simulink model "friction_Pcontrol"  (R2017a)
settings: Solver=ode4  StartTime=0.0  StopTime=80  FixedStep=1e-3  RelTol=1e-3
values from neighbouring files (symbols this model uses):
  ctrl_mass = mass    (= 3.14)    [Script_Friction.m]
  ctrl_ts = 1e-3    (= 0.001)    [Script_Friction.m]
  Fc = 2    [Script_Friction.m]
  Fs = 3    [Script_Friction.m]
  i = 2    [Script_Friction.m]
  kv = 1    [Script_Friction.m]
  m = 3.14    [Static_Identif.m]    (also in static_optim.m)
  mass = 8.1    [C_script_dyn_optimization.m]    (also in Script_Friction.m = 3.14; identify_dynamic_param.m)
  N = 100    [A_Static_Experiment.m]    (also in identify_static_param.m; obtain_sim_data.m = round(length(x) / 2); run_sim.m)
  ref_angle = 0.01    [run_sim.m]
  sigma0 = 1000    [Script_Friction.m]
  sigma1 = 200    [Script_Friction.m]
  sigma2 = 0.1    [C_script_dyn_optimization.m]    (also in Script_Friction.m = 1)
  tol_ss = ref_angle*5e-3    (= 5e-05)    [run_sim.m]
  ts_buffer_stop = ctrl_ts    (= 0.001)    [Script_Friction.m]
  vs = 0.01    [Script_Friction.m]
  X = otim    [A_Static_Experiment.m]    (also in Static_Identif.m = X + 1.0 * V; identify_static_param.m; interval_definition.m = sprintf('Data from interval; static_optim.m = X + 1.0 * V)
undefined symbols (not defined in the file or in its folder): Y, Z
libraries: simulink x11, sm_lib x8, nesl_utility x5, checkpacklib x2, fl_lib x2, Multibody_Multiphysics_Lib x1
settings Model: Creator=jcmonteiro  LastModifiedBy=igricart
settings DataIOCC: ReturnWorkspaceOutputs=on  ReturnWorkspaceOutputsName=SDOSimTest_Log

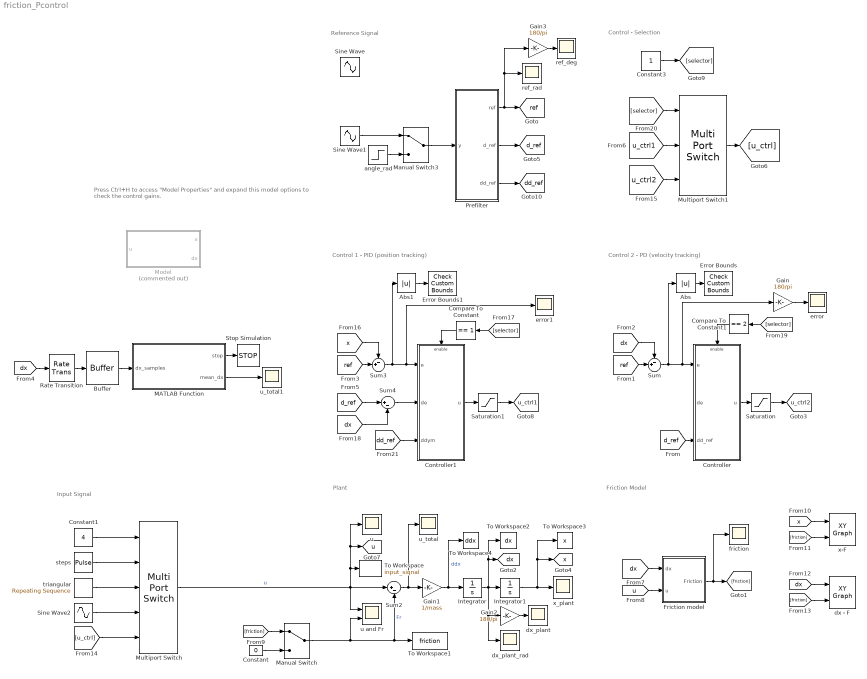
== system friction_Pcontrol ==
  note: Input Signal
  note: Control 2 - PD (velocity tracking)
  note: Plant
  note: Reference Signal
  note: Press Ctrl+H to access "Model Properties" and expand this model options
      | to check the control gains.
  note: Friction Model
  note: Control 1 - PID (position tracking)
  note: Control - Selection
  Abs : Abs
  Abs1 : Abs
  Buffer : Buffer  N=2/ts_buffer_stop  V=2/ts_buffer_stop - 1  ic=(tol_ss + 1) * ones(2/ts_buffer_stop,1)  OutputFrames=off
  Compare To Constant : simulink/Logic and Bit Operations/Compare To Constant  relop===  const=1  OutDataTypeStr=boolean
  Compare To Constant1 : simulink/Logic and Bit Operations/Compare To Constant  relop===  const=2  OutDataTypeStr=boolean
  Constant : Constant  Value=0
  Constant1 : Constant  Value=4
  Constant3 : Constant  OutMin=1  OutMax=2
  Controller : Subsystem  mask{wn=0.5, damp=0.95, far=3}
      mask prompts: wn "Natural frequency"; damp "Damping"; far "Far pole"
      mask init:
      | Kd = far + 2*damp*wn;
      | Kp = wn*wn + 2*damp*wn*far;
      | Ki = far*wn*wn;
  Controller1 : Subsystem  mask{wn=5, damp=0.95, far=2}
      mask prompts: wn "Natural frequency"; damp "Damping"; far "Far pole"
      mask init:
      | Kd = far + 2*damp*wn;
      | Kp = wn*wn + 2*damp*wn*far;
      | Ki = far*wn*wn;
  Error Bounds : checkpacklib/Check Custom Bounds  InstantiateOnLoad=on  enabled=off  stopWhenAssertionFail=off  export=off  ViewDlgPos=[224 43 510 418]  OpenViewOnLoad=off  LaunchViewOnOpen=off  TimeUnits=seconds  EnableUpperBound=on  UpperBoundTimes=[0 1; 1 4; 4 20]  UpperBoundAmplitudes=[4e-3 4e-3; 2e-3 2e-3; 3.5e-4 3.5e-4];  EnableLowerBound=off  LowerBoundTimes=[]  LowerBoundAmplitudes=[]
  Error Bounds1 : checkpacklib/Check Custom Bounds  InstantiateOnLoad=on  enabled=off  stopWhenAssertionFail=off  export=off  ViewDlgPos=[224 43 510 418]  OpenViewOnLoad=off  LaunchViewOnOpen=off  TimeUnits=seconds  EnableUpperBound=on  UpperBoundTimes=[0 1; 1 4; 4 20]  UpperBoundAmplitudes=[4e-3 4e-3; 2e-3 2e-3; 3.5e-4 3.5e-4];  EnableLowerBound=off  LowerBoundTimes=[]  LowerBoundAmplitudes=[]
  Friction model : Subsystem
  Gain : Gain  Gain=180/pi
  Gain1 : Gain  Gain=1/mass
  Gain2 : Gain  Gain=180/pi
  Gain3 : Gain  Gain=180/pi
  Integrator : Integrator
  Integrator1 : Integrator
  MATLAB Function : MATLAB Function  TreatAsAtomicUnit=on
  Manual Switch : ManualSwitch
  Manual Switch3 : ManualSwitch
  Model : Subsystem  Commented=on
  Multiport Switch : MultiPortSwitch  Inputs=4
  Multiport Switch1 : MultiPortSwitch  Inputs=2
  Prefilter : Subsystem  mask{refmodel_wn=6, refmodel_eta=1}
      mask prompts: refmodel_wn "Natural Frequency"; refmodel_eta "Damping"
      mask init:
      | refmodel_eta = abs(refmodel_eta);
      | refmodel_eta = min(refmodel_eta, 1);
      | 
      | refmodel_wn = abs(refmodel_wn);
  Rate Transition : RateTransition  OutPortSampleTime=ts_buffer_stop
  Saturation : Saturate  UpperLimit=20  LowerLimit=-20
  Saturation1 : Saturate  UpperLimit=20  LowerLimit=-20
  Sine Wave : Sin  Amplitude=ref_angle  Frequency=2*pi/1  SampleTime=ctrl_ts
  Sine Wave1 : Sin  Amplitude=0.01  Frequency=2*pi/4  SampleTime=0
  Sine Wave2 : Sin  Amplitude=2.8  Frequency=2*pi  SampleTime=ctrl_ts
  Stop Simulation : Stop
  Sum : Sum  Inputs=-+|
  Sum2 : Sum  Inputs=|+-
  Sum3 : Sum  Inputs=-+|
  Sum4 : Sum  Inputs=|+-
  To Workspace : ToWorkspace  VariableName=input_signal  SaveFormat=Structure With Time  SampleTime=-1
  To Workspace1 : ToWorkspace  VariableName=friction  SaveFormat=Structure With Time  SampleTime=-1
  To Workspace2 : ToWorkspace  VariableName=dx  SaveFormat=Structure With Time  SampleTime=-1
  To Workspace3 : ToWorkspace  VariableName=x  SaveFormat=Structure With Time  SampleTime=-1
  To Workspace4 : ToWorkspace  VariableName=ddx  SaveFormat=Structure With Time  SampleTime=-1
  angle_rad : Step  Time=0  After=ref_angle  SampleTime=0
  dx - F : simulink/Sinks/XY Graph  xmin=-0.6  xmax=0.6  ymin=-Fs*3  ymax=Fs*3  st=-1
  dx_plant : Scope
  dx_plant_rad : Scope
  error : Scope
  error1 : Scope
  friction : Scope
  ref_deg : Scope
  ref_rad : Scope
  steps : DiscretePulseGenerator  PulseType=Time based  Period=10  PulseWidth=5
  triangular : simulink/Sources/Repeating Sequence  rep_seq_t=[0 6]  rep_seq_y=[0 8]
  u : Scope
  u and Fr : Scope  NumInputPorts=2
  u_total : Scope
  u_total1 : Scope
  x-F : simulink/Sinks/XY Graph  xmin=-1e-3  xmax=10e-3  ymin=-Fs*1.2  ymax=Fs*1.2  st=-1
  x_plant : Scope
  tag scope: d_ref=global, dd_ref=global, dx=global, ref=global, u=global, u_ctrl1=global, u_ctrl2=global, x=global
  wires:
  Integrator1/1 -> x_plant/1, To Workspace3/1, [x]
  Integrator/1 -> Gain2/1, dx_plant_rad/1, Integrator1/1, To Workspace2/1, [dx]
  Gain1/1 -> To Workspace4/1, Integrator/1  "ddx"
  Manual Switch3/1 -> Prefilter/1(y)
  angle_rad/1 -> Manual Switch3/2
  Prefilter/1(ref) -> Gain3/1, ref_rad/1, [ref]
  Abs/1 -> Error Bounds/1
  Controller/1(u) -> Saturation/1
  Saturation/1 -> [u_ctrl2]
  Prefilter/2(d_ref) -> [d_ref]
  [d_ref] -> Controller/3(dd_ref)
  Sum/1 -> Abs/1, Gain/1, Controller/1(e)
  [ref] -> Sum/2
  [dx] -> Sum/1
  [dx] -> Friction model/1(dx)
  Sum2/1 -> Gain1/1, u_total/1
  [friction] -> Manual Switch/1
  Constant/1 -> Manual Switch/2
  Manual Switch/1 -> u and Fr/2, To Workspace1/1, Sum2/2  "Fr"
  [friction] -> x-F/2
  [x] -> x-F/1
  [dx] -> dx - F/1
  [friction] -> dx - F/2
  Friction model/1(Friction) -> friction/1, [friction]
  Multiport Switch/1 -> u/1, [u], To Workspace/1, u and Fr/1, Sum2/1  "u"
  Sine Wave1/1 -> Manual Switch3/1
  [u] -> Friction model/2(u)
  [u_ctrl] -> Multiport Switch/5
  Sine Wave2/1 -> Multiport Switch/4
  triangular/1 -> Multiport Switch/3
  steps/1 -> Multiport Switch/2
  Constant1/1 -> Multiport Switch/1
  [d_ref] -> Sum4/1
  [ref] -> Sum3/2
  [dx] -> Sum4/2
  [x] -> Sum3/1
  Controller1/1(u) -> Saturation1/1
  Abs1/1 -> Error Bounds1/1
  Saturation1/1 -> [u_ctrl1]
  Sum4/1 -> Controller1/2(de)
  Sum3/1 -> Abs1/1, error1/1, Controller1/1(e)
  Gain/1 -> error/1
  Gain2/1 -> dx_plant/1
  Gain3/1 -> ref_deg/1
  [dx] -> Rate Transition/1
  Buffer/1 -> MATLAB Function/1(dx_samples)
  MATLAB Function/1(stop) -> Stop Simulation/1
  Rate Transition/1 -> Buffer/1
  MATLAB Function/2(mean_dx) -> u_total1/1
  [u_ctrl1] -> Multiport Switch1/2
  [u_ctrl2] -> Multiport Switch1/3
  [selector] -> Multiport Switch1/1
  Multiport Switch1/1 -> [u_ctrl]
  Constant3/1 -> [selector]
  Compare To Constant/1 -> Controller1/Enable
  Compare To Constant1/1 -> Controller/Enable
  [selector] -> Compare To Constant/1
  [selector] -> Compare To Constant1/1
  Prefilter/3(dd_ref) -> [dd_ref]
  [dd_ref] -> Controller1/3(ddym)

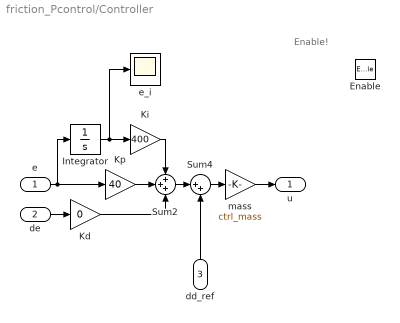
== system friction_Pcontrol/Controller ==
  note: Enable!
  e : Inport  SampleTime=ctrl_ts
  de : Inport  Port=2  SampleTime=ctrl_ts
  dd_ref : Inport  Port=3  SampleTime=ctrl_ts
  Enable : EnablePort
  Integrator : Integrator
  Kd : Gain  Gain=0
  Ki : Gain  Gain=400
  Kp : Gain  Gain=40
  Sum2 : Sum  Inputs=+++
  Sum4 : Sum  Inputs=|++
  e_i : Scope
  mass : Gain  Gain=ctrl_mass
  u : Outport  SampleTime=ctrl_ts
  wires:
  Integrator/1 -> e_i/1, Ki/1
  Sum4/1 -> mass/1
  Ki/1 -> Sum2/1
  de/1 -> Kd/1
  Kd/1 -> Sum2/3
  Kp/1 -> Sum2/2
  mass/1 -> u/1
  e/1 -> Integrator/1, Kp/1
  dd_ref/1 -> Sum4/2
  Sum2/1 -> Sum4/1

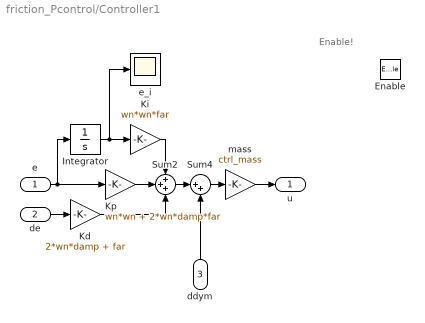
== system friction_Pcontrol/Controller1 ==
  note: Enable!
  e : Inport  SampleTime=ctrl_ts
  de : Inport  Port=2  SampleTime=ctrl_ts
  ddym : Inport  Port=3  SampleTime=ctrl_ts
  Enable : EnablePort
  Integrator : Integrator
  Kd : Gain  Gain=2*wn*damp + far
  Ki : Gain  Gain=wn*wn*far
  Kp : Gain  Gain=wn*wn + 2*wn*damp*far
  Sum2 : Sum  Inputs=+++
  Sum4 : Sum  Inputs=|++
  e_i : Scope
  mass : Gain  Gain=ctrl_mass
  u : Outport  SampleTime=ctrl_ts
  wires:
  Integrator/1 -> e_i/1, Ki/1
  Sum4/1 -> mass/1
  Ki/1 -> Sum2/1
  de/1 -> Kd/1
  Kd/1 -> Sum2/3
  Kp/1 -> Sum2/2
  mass/1 -> u/1
  e/1 -> Integrator/1, Kp/1
  ddym/1 -> Sum4/2
  Sum2/1 -> Sum4/1

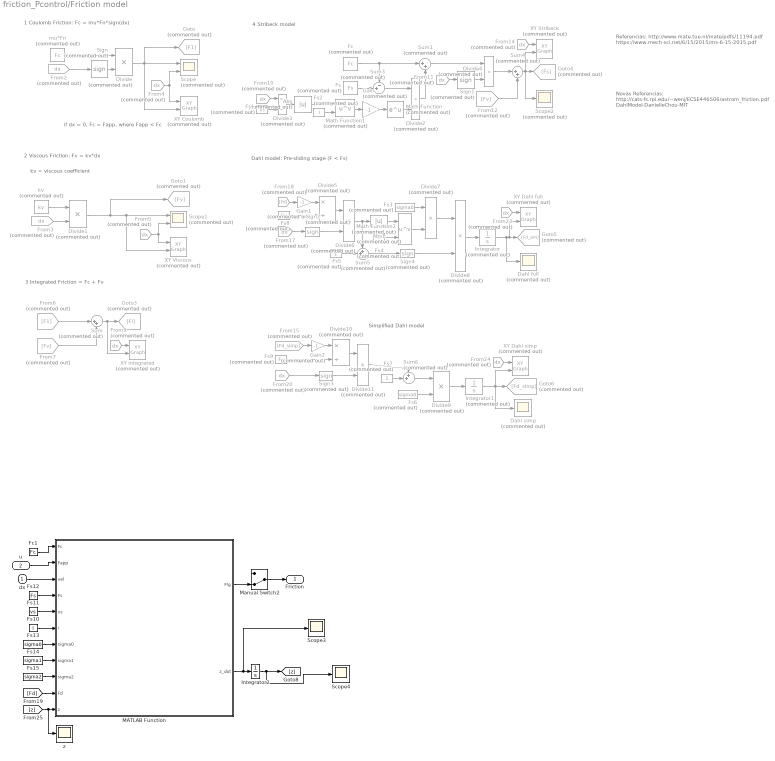
== system friction_Pcontrol/Friction model ==
  note: Novas Referencias:
      | http://cats-fs.rpi.edu/~wenj/ECSE446S06/astrom_friction.pdf
      | DahlModel-DanielleChou-MIT
  note: Simplified Dahl model
  note: Dahl model: Pre-sliding stage (F < Fs)
  note: 4 Stribeck model
  note: 3 Integrated Friction = Fc + Fv
  note: if dx = 0, Fc = Fapp, where Fapp < Fc
  note: kv = viscous coefficient
  note: Referencias:
      | http://www.mate.tue.nl/mate/pdfs/11194.pdf
      | https://www.mech-sci.net/6/15/2015/ms-6-15-2015.pdf
  note: 1 Coulomb Friction: Fc = mu*Fn*sign(dx)
  note: 2 Viscous Friction: Fv = kv*dx
  dx : Inport
  u : Inport  Port=2
  Abs : Abs  Commented=on
  Abs1 : Abs  Commented=on
  Dahl full : Scope  Commented=on
  Dahl simp : Scope  Commented=on
  Divide{,1..2,4,6..9,11} (9 alike) : Product  Commented=on  Inputs=**
  Divide10 : Product  Commented=on  Inputs=*/
  Divide3 : Product  Commented=on  Inputs=*/
  Divide5 : Product  Commented=on  Inputs=*/
  Fc : Constant  Commented=on  Value=Fc
  Fc1 : Constant  Value=Fc
  From{2..5,9..11,14,17,20,23..24} (12 alike) : From  Commented=on  GotoTag=dx
  From12 : From  Commented=on  GotoTag=Fv
  From15 : From  Commented=on  GotoTag=Fd_simp
  From18 : From  Commented=on  GotoTag=Fd
  From6 : From  Commented=on  GotoTag=F1
  From7 : From  Commented=on  GotoTag=Fv
  Fs : Constant  Commented=on  Value=Fs
  Fs1 : Constant  Commented=on  Value=vs
  Fs10 : Constant  Value=i
  Fs11 : Constant  Value=vs
  Fs12 : Constant  Value=Fs
  Fs13 : Constant  Value=sigma0
  Fs14 : Constant  Value=sigma1
  Fs15 : Constant  Value=sigma2
  Fs2 : Constant  Commented=on  Value=i
  Fs3 : Constant  Commented=on  Value=sigma0
  Fs4 : Constant  Commented=on  Value=i
  Fs5 : Constant  Commented=on
  Fs6 : Constant  Commented=on  Value=sigma0
  Fs7 : Constant  Commented=on
  Fs8 : Constant  Commented=on  Value=Fc
  Fs9 : Constant  Commented=on  Value=Fc
  Gain : Gain  Commented=on  Gain=-1
  Gain1 : Gain  Commented=on  Gain=-1
  Gain2 : Gain  Commented=on  Gain=-1
  Goto : Goto  Commented=on  GotoTag=F1
  Goto1 : Goto  Commented=on  GotoTag=Fv
  Goto3 : Goto  Commented=on  GotoTag=Fi
  Goto4 : Goto  Commented=on  GotoTag=Fs
  Goto5 : Goto  Commented=on  GotoTag=Fd_sim
  Goto6 : Goto  Commented=on  GotoTag=Fd_simp
  Integrator : Integrator  Commented=on  InitialCondition=Fc
  Integrator1 : Integrator  Commented=on  InitialCondition=Fc
  Integrator2 : Integrator
  MATLAB Function : MATLAB Function  TreatAsAtomicUnit=on
  Manual Switch2 : ManualSwitch  CurrentSetting=0
  Math Function : Math  Commented=on  SaturateOnIntegerOverflow=on
  Math Function1 : Math  Commented=on  Operator=pow  SaturateOnIntegerOverflow=on
  Math Function2 : Math  Commented=on  Operator=pow  SaturateOnIntegerOverflow=on
  Scope : Scope  Commented=on  NumInputPorts=2
  Scope1 : Scope  Commented=on  NumInputPorts=2
  Scope2 : Scope  Commented=on
  Scope3 : Scope
  Scope4 : Scope
  Sign{,1..4} (5 alike) : Signum  Commented=on
  Sum : Sum  Commented=on  Inputs=|++
  Sum1 : Sum  Commented=on  Inputs=|++
  Sum3 : Sum  Commented=on  Inputs=-+|
  Sum4 : Sum  Commented=on  Inputs=|++
  Sum5 : Sum  Commented=on  Inputs=++|
  Sum6 : Sum  Commented=on  Inputs=++|
  XY Coulomb : simulink/Sinks/XY Graph  Commented=on  xmin=-0.15  xmax=0.15  ymin=-15  ymax=15  st=-1
  XY Dahl full : simulink/Sinks/XY Graph  Commented=on  xmin=-0.2  xmax=0.2  ymin=0  ymax=5  st=-1
  XY Dahl simp : simulink/Sinks/XY Graph  Commented=on  xmin=-0.15  xmax=0.15  ymin=-15  ymax=15  st=-1
  XY Stribeck : simulink/Sinks/XY Graph  Commented=on  xmin=-0.15  xmax=0.15  ymin=-15  ymax=15  st=-1
  XY Viscous : simulink/Sinks/XY Graph  Commented=on  xmin=-0.15  xmax=0.15  ymin=-15  ymax=15  st=-1
  XY integrated : simulink/Sinks/XY Graph  Commented=on  xmin=-0.15  xmax=0.15  ymin=-15  ymax=15  st=-1
  kv : Constant  Commented=on  Value=kv
  mu*Fn : Constant  Commented=on  Value=Fc
  z : Scope
  Friction : Outport
  wires:
  Sign/1 -> Divide/2
  mu*Fn/1 -> Divide/1
  kv/1 -> Divide1/1
  From2/1 -> Sign/1
  Divide1/1 -> XY Viscous/2, Scope1/1, Goto1/1
  From3/1 -> Divide1/2
  Divide/1 -> XY Coulomb/2, Goto/1, Scope/1
  From4/1 -> Scope/2, XY Coulomb/1
  From5/1 -> XY Viscous/1, Scope1/2
  From6/1 -> Sum/1
  From7/1 -> Sum/2
  Sum/1 -> XY integrated/2, Goto3/1
  From9/1 -> XY integrated/1
  Fc/1 -> Sum3/1, Sum1/1
  Fs/1 -> Sum3/2
  Sum3/1 -> Divide2/1
  Math Function/1 -> Divide2/2
  From10/1 -> Divide3/1
  Fs1/1 -> Divide3/2
  Divide3/1 -> Abs/1
  Math Function1/1 -> Gain/1
  Fs2/1 -> Math Function1/2
  Gain/1 -> Math Function/1
  Abs/1 -> Math Function1/1
  Divide2/1 -> Sum1/2
  Sign1/1 -> Divide4/2
  From11/1 -> Sign1/1
  Sum1/1 -> Divide4/1
  Divide4/1 -> Sum4/1
  From12/1 -> Sum4/2
  Sum4/1 -> Scope2/1, XY Stribeck/2, Goto4/1
  From14/1 -> XY Stribeck/1
  From17/1 -> Sign2/1
  Fs8/1 -> Divide5/2
  From18/1 -> Gain1/1
  Gain1/1 -> Divide5/1
  Divide5/1 -> Divide6/1
  Sign2/1 -> Divide6/2
  Divide6/1 -> Sum5/1, Abs1/1
  Fs4/1 -> Math Function2/2
  Abs1/1 -> Math Function2/1
  Math Function2/1 -> Divide7/2
  Fs3/1 -> Divide7/1
  Divide7/1 -> Divide8/1
  Sum5/1 -> Sign4/1
  Divide8/1 -> Integrator/1
  Fs6/1 -> Divide9/2
  Fs5/1 -> Sum5/2
  Divide9/1 -> Integrator1/1
  Fs7/1 -> Sum6/2
  Sum6/1 -> Divide9/1
  Divide11/1 -> Sum6/1
  Sign3/1 -> Divide11/2
  Divide10/1 -> Divide11/1
  Gain2/1 -> Divide10/1
  From15/1 -> Gain2/1
  Fs9/1 -> Divide10/2
  From20/1 -> Sign3/1
  Integrator/1 -> Dahl full/1, XY Dahl full/2, Goto5/1
  From23/1 -> XY Dahl full/1
  From24/1 -> XY Dahl simp/1
  Integrator1/1 -> Dahl simp/1, XY Dahl simp/2, Goto6/1
  Sign4/1 -> Divide8/2
  dx/1 -> MATLAB Function/3(vel)
  Fs10/1 -> MATLAB Function/6(i)
  Fs11/1 -> MATLAB Function/5(vs)
  Fs12/1 -> MATLAB Function/4(Fs)
  Fc1/1 -> MATLAB Function/1(Fc)
  Fs13/1 -> MATLAB Function/7(sigma0)
  [Fd] -> MATLAB Function/10(Fd)
  Integrator2/1 -> Scope4/1, [z]
  MATLAB Function/2(z_dot) -> Scope3/1, Integrator2/1
  Fs14/1 -> MATLAB Function/8(sigma1)
  Fs15/1 -> MATLAB Function/9(sigma2)
  [z] -> z/1, MATLAB Function/11(z)
  MATLAB Function/1(Flg) -> Manual Switch2/2
  Manual Switch2/1 -> Friction/1
  u/1 -> MATLAB Function/2(Fapp)

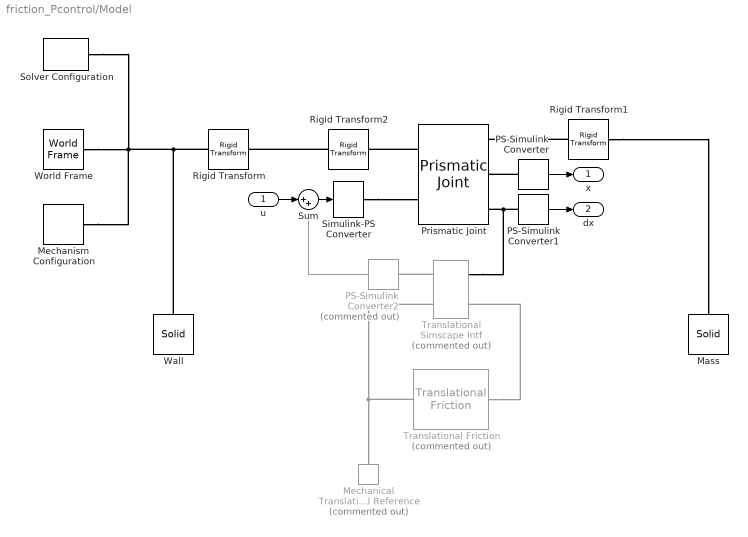
== system friction_Pcontrol/Model ==
  u : Inport
  Mass : sm_lib/Body Elements/Solid  InertiaType=CalculateFromGeometry  Mass=mass  MassUnits=kg  CenterOfMass=[0 0 0]  CenterOfMassUnits=m  MomentsOfInertia=[1 1 1]  MomentsOfInertiaUnits=kg*m^2  ProductsOfInertia=[1 1 1]  ProductsOfInertiaUnits=kg*m^2  DensityBased=off  Density=mass * 1000  DensityUnits=kg/m^3  DoExposeReferenceFrame=on  SerializedFrames=<Frames/>  GraphicType=FromGeometry  MarkerShape=Sphere  MarkerSize=10  GraphicVisPropType=SimpleVisualProperties  GraphicDiffuseColor=[0.5 0.5 0.5]  GraphicSpecularColor=[0.5 0.5 0.5 1.0]  GraphicAmbientColor=[0.15 0.15 0.15 1.0]  GraphicEmissiveColor=[0.0 0.0 0.0 1.0]  GraphicShininess=75  GraphicOpacity=1.0  GeometryShape=Brick  RectangleSize=[1 1]  RectangleSizeUnits=m  BrickDimensions=[10 10 10]  BrickDimensionUnits=cm  CylinderRadius=1  CylinderRadiusUnits=m  CylinderLength=1  CylinderLengthUnits=m  SphereRadius=1  SphereRadiusUnits=m  EllipsoidRadii=[1 1 1]  EllipsoidRadiiUnits=m  ExtrusionCrossSection=[1 1; -1 1; -1 -1; 1 -1]  ExtrusionCrossSectionUnits=m  ExtrusionLength=1  ExtrusionLengthUnits=m  PolygonNumSides=3  PolygonOuterRadius=1  PolygonOuterRadiusUnits=m  ExtGeomFileType=STEP  ExtGeomFileUnits=m  RevolutionCrossSection=[1 1; 1 -1; 2 -1; 2 1]  RevolutionCrossSectionUnits=m  RevolutionExtent=Full  RevolutionAngle=180  RevolutionAngleUnits=deg
  Mechanical Translational Reference : fl_lib/Mechanical/Translational Elements/Mechanical Translational Reference  Commented=on
  Mechanism Configuration : sm_lib/Utilities/Mechanism Configuration  UniformGravity=Constant  GravityVector=[0 0 0]  GravityUnits=m/s^2  LinearizationDelta=0.001
  PS-Simulink Converter : nesl_utility/PS-Simulink Converter  PhysicalDomain=network_engine_domain  SubClassName=ps_output  LeftPortType=input  RightPortType=output  PseudoPeriodic=off  Frequencies=[]  Unit=1  AffineConversion=off
  PS-Simulink Converter1 : nesl_utility/PS-Simulink Converter  PhysicalDomain=network_engine_domain  SubClassName=ps_output  LeftPortType=input  RightPortType=output  PseudoPeriodic=off  Frequencies=[]  Unit=1  AffineConversion=off
  PS-Simulink Converter2 : nesl_utility/PS-Simulink Converter  Commented=on  PhysicalDomain=network_engine_domain  SubClassName=ps_output  LeftPortType=input  RightPortType=output  PseudoPeriodic=off  Frequencies=[]  Unit=N  AffineConversion=off
  Prismatic Joint : sm_lib/Joints/Prismatic Joint  SenseConstraintForce=off  SenseConstraintForceX=off  SenseConstraintForceY=off  SenseConstraintForceZ=off  SenseConstraintTorque=off  SenseConstraintTorqueX=off  SenseConstraintTorqueY=off  SenseConstraintTorqueZ=off  SenseTotalForce=off  SenseTotalForceX=off  SenseTotalForceY=off  SenseTotalForceZ=off  SenseTotalTorque=off  SenseTotalTorqueX=off  SenseTotalTorqueY=off  SenseTotalTorqueZ=off  CompositeWrenchDir=FollowerOnBase  CompositeWrenchFrame=BaseFrame  EquilibriumPosition=0  EquilibriumPositionUnits=m  SpringStiffness=0  SpringStiffnessUnits=N/m  DampingCoefficient=0  DampingCoefficientUnits=N/(m/s)  TorqueActuationMode=InputTorque  MotionActuationMode=ComputedMotion  SensePosition=on  SenseVelocity=on  SenseAcceleration=off  SenseTorqueForce=off  PositionTargetSpecify=off  PositionTargetPriority=High  PositionTargetValue=10  PositionTargetValueUnits=cm  VelocityTargetSpecify=off  VelocityTargetPriority=High  VelocityTargetValue=0  VelocityTargetValueUnits=m/s
  Rigid Transform : sm_lib/Frames and Transforms/Rigid Transform  TranslationMethod=StandardAxis  TranslationStandardOffset=11  TranslationLengthUnit=cm  TranslationStandardAxis=+X  TranslationCartesianOffset=[0 0 0]  TranslationROffset=0  TranslationROffsetUnits=m  TranslationZOffset=0  TranslationZOffsetUnits=m  TranslationThetaOffset=0  TranslationThetaOffsetUnits=deg  RotationMethod=None  RotationAngleUnits=deg  RotationStandardAxis=+Z  RotationAngle=0.0  RotationArbitraryAxis=[0 0 1]  FollAlignAxisA=+X  BaseAlignAxisA=+Y  FollAlignAxisB=+Y  BaseAlignAxisB=+Z  RotationSequenceAxes=FollowerAxes  RotationSequence=XYX  RotationSequenceAngles=[0 0 0]  RotationSequenceAnglesUnits=deg  RotationMatrix=[1 0 0; 0 1 0; 0 0 1]
  Rigid Transform1 : sm_lib/Frames and Transforms/Rigid Transform  TranslationMethod=None  TranslationStandardOffset=11  TranslationLengthUnit=cm  TranslationStandardAxis=+X  TranslationCartesianOffset=[0 0 0]  TranslationROffset=0  TranslationROffsetUnits=m  TranslationZOffset=0  TranslationZOffsetUnits=m  TranslationThetaOffset=0  TranslationThetaOffsetUnits=deg  RotationMethod=AlignedAxes  RotationAngleUnits=deg  RotationStandardAxis=+Z  RotationAngle=0.0  RotationArbitraryAxis=[0 0 1]  FollAlignAxisA=+X  BaseAlignAxisA=+Z  FollAlignAxisB=+Y  BaseAlignAxisB=+X  RotationSequenceAxes=FollowerAxes  RotationSequence=XYX  RotationSequenceAngles=[0 0 0]  RotationSequenceAnglesUnits=deg  RotationMatrix=[1 0 0; 0 1 0; 0 0 1]
  Rigid Transform2 : sm_lib/Frames and Transforms/Rigid Transform  TranslationMethod=None  TranslationStandardOffset=11  TranslationLengthUnit=cm  TranslationStandardAxis=+X  TranslationCartesianOffset=[0 0 0]  TranslationROffset=0  TranslationROffsetUnits=m  TranslationZOffset=0  TranslationZOffsetUnits=m  TranslationThetaOffset=0  TranslationThetaOffsetUnits=deg  RotationMethod=AlignedAxes  RotationAngleUnits=deg  RotationStandardAxis=+Z  RotationAngle=0.0  RotationArbitraryAxis=[0 0 1]  FollAlignAxisA=+Z  BaseAlignAxisA=+X  FollAlignAxisB=+X  BaseAlignAxisB=+Y  RotationSequenceAxes=FollowerAxes  RotationSequence=XYX  RotationSequenceAngles=[0 0 0]  RotationSequenceAnglesUnits=deg  RotationMatrix=[1 0 0; 0 1 0; 0 0 1]
  Simulink-PS Converter : nesl_utility/Simulink-PS Converter  PhysicalDomain=network_engine_domain  SubClassName=ps_input  LeftPortType=input  RightPortType=output  PseudoPeriodic=off  Frequencies=[]  NoiseDistribution=none  NoiseParameters=[]  Unit=N  AffineConversion=off  FilteringAndDerivatives=zero  SimscapeFilterOrder=1  InputFilterTimeConstant=0.001  UdotUserProvided=1
  Solver Configuration : nesl_utility/Solver Configuration  PhysicalDomain=network_engine_domain  SubClassName=solver  LeftPortType=input  RightPortType=generic  Accelerate=off  Tones=[]  Harmonics=[]  SimulateNoise=off  Profile=off  UseLocalSampling=off  EnableSwitchedLinearOptims=on  FrequencyDomain=off  UseCCode=off  RelTol=0.001  AbsTol=1e-06  MinStep=1e-09  ToWorkspace=off  RevertToSquareIcSolve=off  NumHomotopyIterations=100  PhasorMode=off  PhasorModeNumHarmonics=1  OverrideAbsTol=off  DoDC=on  ResidualTolerance=1e-09  UseLocalSolver=off  LocalSolverChoice=NE_BACKWARD_EULER_ADVANCER  LocalSolverSampleTime=0.001  DoFixedCost=off  MaxNonlinIter=3  MaxModeIter=2  LinearAlgebra=Sparse  DelaysMemoryBudget=1024  AutomaticFiltering=on  FilteringTimeConstant=0.001
  Sum : Sum  Inputs=|++
  Translational Friction : fl_lib/Mechanical/Translational Elements/Translational Friction  Commented=on  brkwy_frc=0.8 N  brkwy_vel=deg2rad(0.5) m/s  Col_frc=0.7 N  visc_coef=0 N/(m/s)  v_specify=off  v_priority=High  v=0 m/s  v_nominal_specify=off  v_nominal_unit=m/s  v_nominal_value=1  f_specify=off  f_priority=None  f=0 N  f_nominal_specify=off  f_nominal_unit=N  f_nominal_value=1
      settings: SourceProductName=Simscape  SourceProductBaseCode=SS
  Translational Simscape Intf : Multibody_Multiphysics_Lib/Interfaces/Translational Simscape Intf  Commented=on
      settings: SourceProductName=Simscape Multibody Multiphysics Library
  Wall : sm_lib/Body Elements/Solid  InertiaType=CalculateFromGeometry  Mass=1  MassUnits=kg  CenterOfMass=[0 0 0]  CenterOfMassUnits=m  MomentsOfInertia=[1 1 1]  MomentsOfInertiaUnits=kg*m^2  ProductsOfInertia=[1 1 1]  ProductsOfInertiaUnits=kg*m^2  DensityBased=on  Density=1000  DensityUnits=kg/m^3  DoExposeReferenceFrame=on  SerializedFrames=<Frames/>  GraphicType=FromGeometry  MarkerShape=Sphere  MarkerSize=10  GraphicVisPropType=SimpleVisualProperties  GraphicDiffuseColor=[0.5 0.5 0.5]  GraphicSpecularColor=[0.5 0.5 0.5 1.0]  GraphicAmbientColor=[0.15 0.15 0.15 1.0]  GraphicEmissiveColor=[0.0 0.0 0.0 1.0]  GraphicShininess=75  GraphicOpacity=1.0  GeometryShape=Brick  RectangleSize=[1 1]  RectangleSizeUnits=m  BrickDimensions=[1 100 100]  BrickDimensionUnits=cm  CylinderRadius=1  CylinderRadiusUnits=m  CylinderLength=1  CylinderLengthUnits=m  SphereRadius=1  SphereRadiusUnits=m  EllipsoidRadii=[1 1 1]  EllipsoidRadiiUnits=m  ExtrusionCrossSection=[1 1; -1 1; -1 -1; 1 -1]  ExtrusionCrossSectionUnits=m  ExtrusionLength=1  ExtrusionLengthUnits=m  PolygonNumSides=3  PolygonOuterRadius=1  PolygonOuterRadiusUnits=m  ExtGeomFileType=STEP  ExtGeomFileUnits=m  RevolutionCrossSection=[1 1; 1 -1; 2 -1; 2 1]  RevolutionCrossSectionUnits=m  RevolutionExtent=Full  RevolutionAngle=180  RevolutionAngleUnits=deg
  World Frame : sm_lib/Frames and Transforms/World Frame
  x : Outport
  dx : Outport  Port=2
  wires:
  u/1 -> Sum/1
  PS-Simulink Converter/1 -> x/1
  PS-Simulink Converter1/1 -> dx/1
  PS-Simulink Converter2/1 -> ?
  Sum/1 -> Simulink-PS Converter/1
  connections:
  Simulink-PS Converter/RConn1 -- Prismatic Joint/LConn2
  Wall/RConn1 -- Rigid Transform/LConn1 -- Solver Configuration/RConn1 -- Mechanism Configuration/RConn1 -- World Frame/RConn1
  Rigid Transform2/LConn1 -- Rigid Transform/RConn1
  Rigid Transform1/RConn1 -- Mass/RConn1
  Rigid Transform1/LConn1 -- Prismatic Joint/RConn1
  Prismatic Joint/LConn1 -- Rigid Transform2/RConn1
  PS-Simulink Converter/LConn1 -- Prismatic Joint/RConn2
  PS-Simulink Converter1/LConn1 -- Translational Simscape Intf/RConn1 -- Prismatic Joint/RConn3
  Translational Friction/RConn1 -- Mechanical Translational Reference/LConn1 -- Translational Simscape Intf/LConn2
  Translational Friction/LConn1 -- Translational Simscape Intf/RConn2
  Translational Simscape Intf/LConn1 -- PS-Simulink Converter2/LConn1

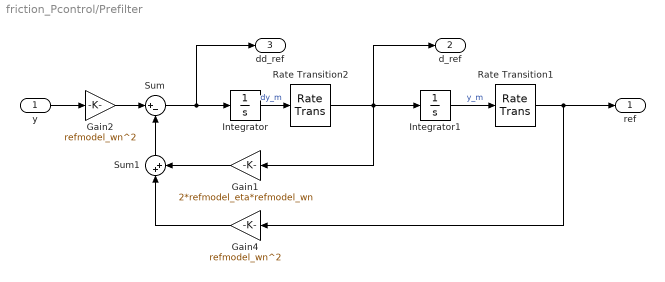
== system friction_Pcontrol/Prefilter ==
  y : Inport
  Gain1 : Gain  Gain=2*refmodel_eta*refmodel_wn
  Gain2 : Gain  Gain=refmodel_wn^2
  Gain4 : Gain  Gain=refmodel_wn^2
  Integrator : Integrator
  Integrator1 : Integrator
  Rate Transition1 : RateTransition  OutPortSampleTime=ctrl_ts
  Rate Transition2 : RateTransition  OutPortSampleTime=ctrl_ts
  Sum : Sum  Inputs=|+-
  Sum1 : Sum  Inputs=|++
  ref : Outport
  d_ref : Outport  Port=2
  dd_ref : Outport  Port=3
  wires:
  Sum/1 -> Integrator/1, dd_ref/1
  Integrator/1 -> Rate Transition2/1  "dy_m"
  Integrator1/1 -> Rate Transition1/1  "y_m"
  Gain4/1 -> Sum1/1
  Gain2/1 -> Sum/1
  y/1 -> Gain2/1
  Gain1/1 -> Sum1/2
  Sum1/1 -> Sum/2
  Rate Transition2/1 -> Gain1/1, Integrator1/1, d_ref/1
  Rate Transition1/1 -> ref/1, Gain4/1

== matlab function friction_Pcontrol/MATLAB Function ==
  data: dx_samples input; stop output; tol_ss parameter; mean_dx output
function [stop, mean_dx]= stop_criterion(dx_samples, tol_ss)
    mean_dx = mean(dx_samples);
    stop = max( abs(dx_samples - mean_dx) ) < tol_ss;
end

== matlab function friction_Pcontrol/Friction model/MATLAB Function ==
  data: Fc input; Fapp input; vel input; Fs input; vs input; i input; sigma0 input; sigma1 input; sigma2 input; Fd input; Flg output; z_dot output; z input
%% Function with friction models

function [Flg ,z_dot] = friction(Fc ,Fapp ,vel ,Fs ,vs ,i ,sigma0 ,sigma1 ,sigma2 ,Fd ,z)

%% Coulomb Friction and Viscous Friction
% if vel ~= 0
%     Fcoulomb = Fc*sign(vel);
%     Fv = sigma2*vel + Fcoulomb;
% elseif abs(Fapp) < Fs
%     Fcoulomb = Fapp;
%     Fv = Fcoulomb;
% else %v == 0 && abs(Fapp) >= Fs
%     Fcoulomb = Fc*sign(Fapp);
%     Fv = Fcoulomb;
% end
   
%% Integrated Coulomb Friction and Viscous Friction with friction force
% transition
% if (vel >= 0)
%     Fi = min(Fc,Fv);
% else
%     Fi = max(-Fc,Fv);
% end

%% Stribeck model
% F = (Fc + (Fs - Fc) * exp(-(abs(vel/vs))^i)) * sign(vel) + Fv;
% 
% if vel ~= 0
%     Fstrib = F;
% elseif abs(Fapp) < Fs
%     Fstrib = Fapp;
% else %v == 0 && abs(Fapp) >= Fs
%     Fstrib = Fs*sign(Fapp);
% end

%% Dahl Model - Pre-sliding (Fd < Fs)
% % d_Fd_dx = sigma0 * (abs(1 - Fd/Fc * sign(vel)))^i * sign(1 - Fd / Fc * sign(vel));
% d_Fd_dx = sigma0 * (abs(1 - Fd/Fc * sign(vel)))^i;
% 
% %Simplified model where i = 1
% %d_Fd_dx_mod = sigma0 * (1 - Fd/Fc * sign(vel));
% 
% % OBs.: d_Fd_dt  = d_Fd_dx * dx_dt
% d_Fd_dt = d_Fd_dx * vel;

%% LuGre model
% Alpeter dc thesis
% Normally i  =  2
g_xdot = Fc + (Fs - Fc) * exp(-(abs(vel/vs))^i);
% z_dot = vel - sigma0 * vel * z / g_xdot;
% Flg = sigma0 * z + sigma1 * z_dot + sigma2 * vel;

%Astrom paper
% Variable damping coefficient decreasing with increasing velocity
vd = 1e-1; 
sigma1_v = sigma1*exp(-(vel/vd)^2);

% Olsson paper
% g_xdot = Fc + (Fs - Fc) * exp(-i*abs(vel));
z_dot = vel - sigma0 * abs(vel) * z / g_xdot;
Flg = sigma0 * z + sigma1 * z_dot + sigma2 * vel;
